simulink model "ControlSystem"  (R2024b)
settings: Solver=FixedStepAuto  StartTime=0.0  StopTime=80  RelTol=1e-3  EnableMultiTasking=on
values from neighbouring files (symbols this model uses):
  A_ESO_d = [1-l1_ESO_d, delta_t-l1_ESO_d*delta_t, 1/2 * delta_t^2 - 1/2 * l1_ESO_d*delta_t^2 ... (first row only)    [ControlSystem_Vars.m]
  A_kalman = [1 delta_t ... (first row only)    [AttitudePlayground_Vars.m]    (also in ControlSystem_Vars.m)
  A_MESO_d = A_o_d - l_MESO_d*C_o_d*A_o_d    [ControlSystem_Vars.m]
  A_O_d = A_m_dlqr - l_o_d*c_m_dlqr*A_m_dlqr    [ControlSystem_Vars.m]
  acc_sigma = 0.2 * calc_sigma(acc_pp)    [AttitudePlayground_Vars.m]    (also in ControlSystem_Vars.m)
  amfitrack_time = 1    [ControlSystem_Vars.m]
  b0 = 1.025    [ControlSystem_Vars.m]
  b_ESO_d = [1/2*b0*delta_t^2 - l1_ESO_d*b0*delta_t^2 ... (first row only)    [ControlSystem_Vars.m]
  B_MESO_d = B_o_d - l_MESO_d*C_o_d*B_o_d    [ControlSystem_Vars.m]
  B_O_d = b_m_dlqr - l_o_d*c_m_dlqr*b_m_dlqr    [ControlSystem_Vars.m]
  C_kalman = eye(2)    [AttitudePlayground_Vars.m]    (also in ControlSystem_Vars.m)
  delta_t = 0.01    [AttitudePlayground_Vars.m]    (also in ControlSystem_Vars.m; ParameterIdentification.m = t2 - t1)
  DLADRC_max_effort = 100-motor_bias    (= 70)    [ControlSystem_Vars.m]
  DLQR_ADRCNM_max_effort = 100-motor_bias    (= 70)    [ControlSystem_Vars.m]
  DLQR_max_effort = 100-motor_bias    (= 70)    [ControlSystem_Vars.m]
  DLQRMADRC_max_effort = 100-motor_bias    (= 70)    [ControlSystem_Vars.m]
  gyro_sigma_3d = [1*gyro_sigma, 1*gyro_sigma, gyro_sigma]    [AttitudePlayground_Vars.m]    (also in ControlSystem_Vars.m)
  k1_c_d = (1 - z_cl)^2/delta_t^2    [ControlSystem_Vars.m]
  k_c_T_dlqr = dlqr(A_m_dlqr,b_m_dlqr,Q,R)    [ControlSystem_Vars.m]
  k_d_T_dlqr_adrcnm = k_d_T_lqr    [ControlSystem_Vars.m]
  k_d_T_lqr = (e_m*c_T_d_m_lqr)\b_m_lqr    [ControlSystem_Vars.m]
  k_dlqr = k_c_T_dlqr    [ControlSystem_Vars.m]
  k_dlqr_adrcnm = dlqr(A_dlqr_adrcnm,B_dlqr_adrcnm,Q,R)    [ControlSystem_Vars.m]
  k_s_dlqr = -inv(c_T_m_lqr*inv(A_m_lqr-b_m_lqr*k_c_T_dlqr)*b_m_lqr)    [ControlSystem_Vars.m]
  k_T_d = [k1_c_d, k2_c_d]    [ControlSystem_Vars.m]
  l_ESO_d = [l1_ESO_d, l2_ESO_d, l3_ESO_d]'    [ControlSystem_Vars.m]
  l_MESO_d = acker(A_o_d',C_o_d',[z_MESO,z_MESO,z_MESO])'    [ControlSystem_Vars.m]
  l_o_d = acker(A_m_dlqr',c_m_dlqr',[z_o,z_o])'    [ControlSystem_Vars.m]
  motor_bias = 30    [ControlSystem_Vars.m]
  N = 1    [AttitudePlayground_Vars.m]    (also in ControlSystem_Vars.m = 2)
  P_0 = eye(4)    [AttitudePlayground_Vars.m]    (also in ControlSystem_Vars.m)
  q_sigma = 0.001    [AttitudePlayground_Vars.m]    (also in ControlSystem_Vars.m)
  R_kalman = diag([(calc_sigma(0.8))^2, (0.07)^2])    [AttitudePlayground_Vars.m]    (also in ControlSystem_Vars.m)
  reset_time = 20    [ControlSystem_Vars.m]
undefined symbols (not defined in the file or in its folder): Discrete, Time
libraries: simulink_extras x6, bbblueActuatorLib x4, ctrlSharedLib x1, bbblueSensorLib x1, sharedutil x1, dspstat3 x1, bbblueCommlib x1
settings Model: ExtModeTrigDuration=100  Creator=Henrik  LastModifiedBy=Henrik
settings SolverCC: PositivePriorityOrder=on
settings OptimizationCC: DefaultParameterBehavior=Inlined  EnhancedBackFolding=on  PassReuseOutputArgsAs=Individual arguments  ZeroExternalMemoryAtStartup=off  ZeroInternalMemoryAtStartup=off  MaxStackSize=64  OptimizeBlockOrder=speed  DifferentSizesBufferReuse=on  OptimizationCustomize=off  EfficientTunableParamExpr=on
settings DebuggingCC: ParameterTunabilityLossMsg=error
settings HardwareCC: ProdBitPerPointer=32  ProdBitPerSizeT=32  ProdBitPerPtrDiffT=32  ProdLargestAtomicInteger=Long  ProdLargestAtomicFloat=Double  ProdWordSize=32  ProdHWDeviceType=ARM Compatible->ARM Cortex-A (32-bit)  UseEmbeddedCoderFeatures=off
settings SFSimCC: MATLABDynamicMemAlloc=off
settings RTWCC: Description=Embedded Coder  SystemTargetFile=ert.tlc  HardwareBoard=BeagleBone Blue  TLCOptions="-aInlineSetEventsForThisBaseRateFcn=TLC_FALSE -aSuppressMultiTaskScheduler=TLC_FALSE  -aRateBasedStepFcn=0"  TemplateMakefile=ert_default_tmf  Toolchain=GNU GCC BeagleBone Blue
settings CodeAppCC: ForceParamTrailComments=on  IgnoreCustomStorageClasses=off  OperatorAnnotations=on  SimulinkDataObjDesc=on  SFDataObjDesc=on  InsertBlockDesc=on
settings ERTTargetCC: SupportNonInlinedSFcns=on  SupportVariableSizeSignals=on

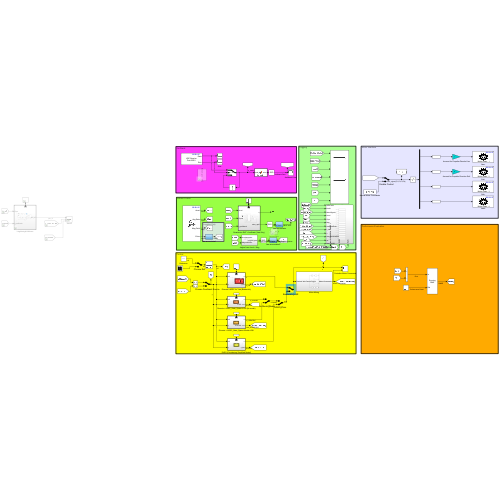
[thumbnail: Simulink's stored preview of the top-level diagram]
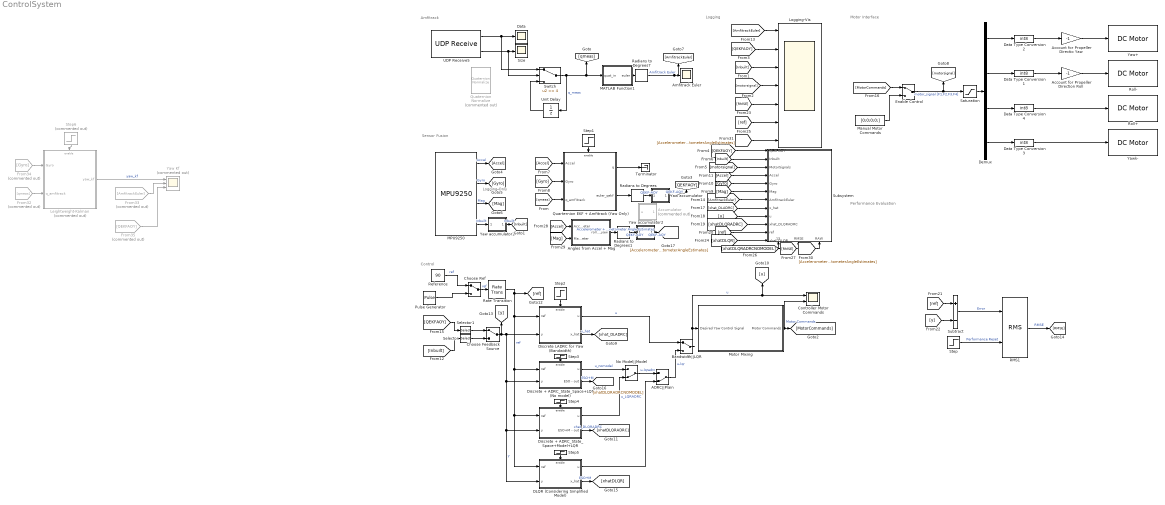
== system ControlSystem ==
  note: Performance Evaluation
  note: Control
  note: Logging Only
  note: Logging
  note: Sensor Fusion
  note: Amfitrack
  note: Motor Interface
  ADRC||Plain : ManualSwitch  CurrentSetting=0
  Account for Propeller Directio Yaw : Gain  Gain=-1  OutDataTypeStr=int8
  Account for Propeller Direction Roll : Gain  Gain=-1  OutDataTypeStr=int8
  Accumulator : Subsystem  Commented=on
  Amfitrack Euler : Scope
  Angles from Accel + Mag : Subsystem
  Bandwidth||LQR : ManualSwitch
  Choose Feedback Source : ManualSwitch
  Choose Ref : ManualSwitch
  Controller Motor Commands : Scope  NumInputPorts=2
  DLQR (Considering Simplified Model) : Subsystem
  Data : Scope
  Data Type Conversion{1..4} (4 alike) : DataTypeConversion  OutDataTypeStr=int8  SaturateOnIntegerOverflow=off  RndMeth=Floor
  Demux : Demux
  Discrete + ADRC_State_Space+LQR (No model) : Subsystem
  Discrete + ADRC_State_Space+Model+LQR : Subsystem
  Discrete LADRC for Yaw (Bandwidth) : Subsystem
  Enable Control : ManualSwitch
  From32 : From  Commented=on  GotoTag=qmeas
  From33 : From  Commented=on  GotoTag=AmfitrackEuler
  From34 : From  Commented=on  GotoTag=Gyro
  From35 : From  Commented=on  GotoTag=QEKFAOY
  Leightweight-Kalman : Subsystem  Commented=on
  Logging-Vis : Scope  NumInputPorts=7
  MATLAB Function1 : MATLAB Function  TreatAsAtomicUnit=on
  MPU9250 : bbblueSensorLib/MPU9250  OperationMode=DMP  Accel=on  AngularRate=on  Ak8963Field=on  EulerAngles=on  Quat=off  AccelRange=2G  Acceldlpf=1  GyroRange=250 dps  Gyrodlpf=1  DmpOdr=200 Hz  SampleTime=delta_t
  Manual Motor Commands : Constant  Value=[0;0;0;0;]
  Motor Mixing : Subsystem
  No Model||Model : ManualSwitch  CurrentSetting=0
  Pulse Generator : DiscretePulseGenerator  PulseType=Time based  Amplitude=90  Period=40  PulseWidth=50  PhaseDelay=25
  Quarternion EKF + Amfitrack (Yaw Only) : Subsystem
  Quaternion Normalize : sharedutil/Quaternion Normalize  Commented=on  aMode=aMode
  RMS1 : dspstat3/RMS  run=on  directionMode=Each column  dimension=1  reset_popup=Rising edge
  Radians to Degrees : simulink_extras/Transformations/Radians to Degrees
  Radians to Degrees1 : simulink_extras/Transformations/Radians to Degrees
  Radians to Degrees7 : simulink_extras/Transformations/Radians to Degrees
  Rate Transition : RateTransition  OutPortSampleTime=delta_t
  Reference : Constant  Value=90
  Roll+ : bbblueActuatorLib/DC Motor  index=3  stopaction=Free Spin  SimulateUsing=Code generation
  Roll- : bbblueActuatorLib/DC Motor  index=2  stopaction=Free Spin  SimulateUsing=Code generation
  Saturation : Saturate  UpperLimit=motor_bias + DLADRC_max_effort  LowerLimit=0
  Selector : Selector  InputPortWidth=3  IndexOptions=Index vector (dialog)  Indices=[3]  OutputSizes=1
  Selector1 : Selector  InputPortWidth=3  IndexOptions=Index vector (dialog)  Indices=[3]  OutputSizes=1
  Size : Scope
  Step : Step  Time=reset_time  SampleTime=delta_t
  Step{1..5} (5 alike) : Step  Time=amfitrack_time  SampleTime=delta_t
  Step6 : Step  Commented=on  Time=amfitrack_time  SampleTime=delta_t
  Subsystem : Subsystem
      settings: PortSchema="{\"entries\":[{\"content\":{\"sides\":[{\"content\":{\"connectorIds\":[\"In1\",\"In2\",\"In3\",\"In4\",\"In5\",\"In6\",\"In7\",\"In8\",\"In9\",\"In10\",\"In11\",\"In12\"]},\"type\":\"ConnectorPlacement.EquallySpacedRectSide\",\"uuid\":\"991a5da0-df7a-4ef3-96ef-0456b705c574\"},{\"content\":{\"side\":\"RIGHT\"},\"type\":\"ConnectorPlacement.EquallySpacedRectSide\",\"uuid\":\"461993a6-f70f-45cb-8f04-a275f01d98e3\"},{\"content\":{\"side\":\"TOP\"},\"type\":\"ConnectorPlacement.EquallySpacedRectSide\",\"uuid\":\"99c0c584-10a5-4b90-9562-b870c5806d76\"},{\"content\":{\"connectorIds\":[\"In13\",\"In14\",\"In15\"],\"side\":\"BOTTOM\"},\"type\":\"ConnectorPlacement.EquallySpacedRectSide\",\"uuid\":\"fd03c8b6-ebae-4f62-b996-a229c9f073bc\"}]},\"type\":\"ConnectorPlacement.EquallySpacedConnector\",\"uuid\":\"7a0ee6bb-fc46-401d-998f-74e037bdb036\"}],\"packageUris\":[\"http://schema.mathworks.com/mf0/Connector/R2020b\"],\"version\":\"1.0\"}"
  Subtract : Sum  Inputs=+-
  Switch : Switch  Threshold=4  SaturateOnIntegerOverflow=off  InputSameDT=off
  Terminator : Terminator
  UDP Receive5 : bbblueCommlib/UDP Receive  localURL='0.0.0.0'  localPort=25001  remoteURL='0.0.0.0'  remotePort=-1  recvBufferSize=8192  signalDatatype=double  dims=4  isVarSize=off  showBlockingTime=off  blockingTime=0  sampletime=delta_t  blockPlatform=BB BLUE
  Unit Delay : UnitDelay  InitialCondition=[1,0,0,0]'  SampleTime=-1  HasFrameUpgradeWarning=on
  Yaw Kf : Scope  Commented=on  NumInputPorts=3
  Yaw accumulator : Subsystem
  Yaw accumulator1 : Subsystem
  Yaw accumulator2 : Subsystem
  Yaw+ : bbblueActuatorLib/DC Motor  index=1  stopaction=Free Spin  SimulateUsing=Code generation
  Yawk- : bbblueActuatorLib/DC Motor  index=4  stopaction=Free Spin  SimulateUsing=Code generation
  wires:
  Unit Delay/1 -> Switch/3
  UDP Receive5/2 -> Switch/2, Size/1
  UDP Receive5/1 -> Switch/1, Data/1
  MATLAB Function1/1(euler) -> Radians to Degrees7/1
  Radians to Degrees7/1 -> Amfitrack Euler/1, [AmfitrackEuler]  "Amfitrack Euler"
  Switch/1 -> MATLAB Function1/1(quat_in), [qmeas], Unit Delay/1  "q_meas"
  [qmeas] -> Quarternion EKF + Amfitrack (Yaw Only)/3(q_amfitrack)
  Quarternion EKF + Amfitrack (Yaw Only)/1(q) -> Terminator/1
  Yaw accumulator/1(yaw_acc) -> [QEKFAOY]  "QEKF-AOY"
  [Inbuilt] -> Logging-Vis/3
  [motorsignal] -> Logging-Vis/4
  [QEKFAOY] -> Logging-Vis/2
  MPU9250/4 -> Yaw accumulator1/1(yaw)  "Inbuilt"
  MPU9250/3 -> [Mag]  "Mag"
  MPU9250/1 -> [Accel]  "Accel"
  [Accel] -> Quarternion EKF + Amfitrack (Yaw Only)/1(Accel)
  MPU9250/2 -> [Gyro]  "Gyro"
  [Gyro] -> Quarternion EKF + Amfitrack (Yaw Only)/2(Gyro)
  [QEKFAOY] -> Subsystem/1(QEKFAOY)
  [motorsignal] -> Subsystem/3(MotorSignals)
  [Inbuilt] -> Subsystem/2(Inbuilt)
  [Mag] -> Subsystem/6(Mag)
  [Gyro] -> Subsystem/5(Gyro)
  [Accel] -> Subsystem/4(Accel)
  [AmfitrackEuler] -> Logging-Vis/1
  [AmfitrackEuler] -> Subsystem/7(AmfitrackEuler)
  Account for Propeller Directio Yaw/1 -> Yaw+/1
  Data Type Conversion2/1 -> Account for Propeller Directio Yaw/1
  Data Type Conversion3/1 -> Yawk-/1
  Demux/1 -> Data Type Conversion2/1
  Demux/4 -> Data Type Conversion3/1
  Account for Propeller Direction Roll/1 -> Roll-/1
  Data Type Conversion1/1 -> Account for Propeller Direction Roll/1
  Demux/2 -> Data Type Conversion1/1
  Demux/3 -> Data Type Conversion4/1
  Data Type Conversion4/1 -> Roll+/1
  Saturation/1 -> Demux/1
  Enable Control/1 -> Saturation/1, [motorsignal]  "motor_signal [F1,F2,F3,F4]"
  Quarternion EKF + Amfitrack (Yaw Only)/2(euler_qekf) -> Radians to Degrees/1
  Manual Motor Commands/1 -> Enable Control/2
  Radians to Degrees/1 -> Yaw accumulator/1(yaw)  "QEKF-AOY"
  Yaw accumulator1/1(yaw_acc) -> [Inbuilt]  "Inbuilt"
  Bandwidth||LQR/1 -> [u], Controller Motor Commands/1, Motor Mixing/1(Desired Yaw Control Signal)  "u"
  Choose Feedback Source/1 -> DLQR (Considering Simplified Model)/2(y), Discrete + ADRC_State_Space+Model+LQR/2(y), Discrete + ADRC_State_Space+LQR (No model)/2(y), Discrete LADRC for Yaw (Bandwidth)/2(y), [y]  "y"
  Selector/1 -> Choose Feedback Source/2
  Selector1/1 -> Choose Feedback Source/1
  [Inbuilt] -> Selector/1
  [QEKFAOY] -> Selector1/1
  Rate Transition/1 -> [ref], Discrete + ADRC_State_Space+LQR (No model)/1(ref), DLQR (Considering Simplified Model)/1(ref), Discrete + ADRC_State_Space+Model+LQR/1(ref), Discrete LADRC for Yaw (Bandwidth)/1(ref)  "ref"
  Motor Mixing/1(Motor Commands) -> Controller Motor Commands/2, [MotorCommands]  "Motor Commands"
  [MotorCommands] -> Enable Control/1
  Discrete LADRC for Yaw (Bandwidth)/2(x_hat) -> [xhat_DLADRC]  "x_hat"
  [xhat_DLADRC] -> Subsystem/8(x_hat)
  [u] -> Subsystem/9(u)
  ADRC||Plain/1 -> Bandwidth||LQR/2  "u-lqr"
  Discrete LADRC for Yaw (Bandwidth)/1(u) -> Bandwidth||LQR/1  "u"
  Discrete + ADRC_State_Space+Model+LQR/2(ESO+M - out) -> [xhatDLQRADRC]  "xhat_DLQRADRC"
  [xhatDLQRADRC] -> Subsystem/10(xhat_DLQRADRC)
  [ref] -> Subsystem/11(ref)
  Subtract/1 -> RMS1/1  "Error"
  Step/1 -> RMS1/2  "Performance Reset"
  [ref] -> Subtract/1
  [y] -> Subtract/2
  RMS1/1 -> [RMSE]  "RMSE"
  [RMSE] -> Logging-Vis/5
  DLQR (Considering Simplified Model)/2(x_hat) -> [xhatDLQR]  "ESO+M"
  Discrete + ADRC_State_Space+Model+LQR/1(u) -> No Model||Model/2  "u_LQRADRC"
  DLQR (Considering Simplified Model)/1(u) -> ADRC||Plain/2
  [xhatDLQR] -> Subsystem/12(xhat_DLQR)
  Reference/1 -> Choose Ref/1  "ref"
  [ref] -> Logging-Vis/6
  Pulse Generator/1 -> Choose Ref/2
  Choose Ref/1 -> Rate Transition/1  "ref"
  Discrete + ADRC_State_Space+LQR (No model)/1(u) -> No Model||Model/1  "u_nomodel"
  No Model||Model/1 -> ADRC||Plain/1  "u-lqradrc"
  Discrete + ADRC_State_Space+LQR (No model)/2(ESO - out) -> [xhatDLQRADRCNOMODEL]  "ESO+M"
  [xhatDLQRADRCNOMODEL] -> Subsystem/13(xhatDLQRADRCNOMODEL)
  [RMSE] -> Subsystem/14(RMSE)
  [Accel] -> Angles from Accel + Mag/1(Accelerometer)
  [Mag] -> Angles from Accel + Mag/2(Magnetometer)
  Angles from Accel + Mag/1(roll,pitch,yaw) -> Radians to Degrees1/1  "Accelerometer + Magnetometer Angle Estimates"
  [AccelerometerMagnetometerAngleEstimates] -> Subsystem/15(RAW)
  [AccelerometerMagnetometerAngleEstimates] -> Logging-Vis/7
  Radians to Degrees1/1 -> Yaw accumulator2/1(yaw)  "QEKF-AOY"
  Yaw accumulator2/1(yaw_acc) -> [AccelerometerMagnetometerAngleEstimates]  "QEKF-AOY"
  Step1/1 -> Quarternion EKF + Amfitrack (Yaw Only)/Enable
  Step2/1 -> Discrete LADRC for Yaw (Bandwidth)/Enable
  Step3/1 -> Discrete + ADRC_State_Space+LQR (No model)/Enable
  Step4/1 -> Discrete + ADRC_State_Space+Model+LQR/Enable
  Step5/1 -> DLQR (Considering Simplified Model)/Enable
  From34/1 -> Leightweight-Kalman/1(Gyro)
  Step6/1 -> Leightweight-Kalman/Enable
  Leightweight-Kalman/1(yaw_kf) -> Yaw Kf/1  "yaw_kf"
  From32/1 -> Leightweight-Kalman/2(q_amfitrack)
  From33/1 -> Yaw Kf/2
  From35/1 -> Yaw Kf/3

== system ControlSystem/Accumulator ==
  u : Inport
  MATLAB Function : MATLAB Function  TreatAsAtomicUnit=on
  Unit Delay1 : UnitDelay  SampleTime=-1  HasFrameUpgradeWarning=on
  Unit Delay2 : UnitDelay  SampleTime=-1  HasFrameUpgradeWarning=on
  u_cul : Outport
  wires:
  u/1 -> Unit Delay1/1, MATLAB Function/1(u)
  Unit Delay1/1 -> MATLAB Function/2(u_prev)
  Unit Delay2/1 -> MATLAB Function/3(u_cul_prev)
  MATLAB Function/1(u_cul) -> u_cul/1, Unit Delay2/1  "u_cul"

== system ControlSystem/Angles from Accel + Mag ==
  Accelerometer : Inport
  Magnetometer : Inport  Port=2
  Demux : Demux  Outputs=3
  Demux2 : Demux  Outputs=3
  MATLAB Function : MATLAB Function  TreatAsAtomicUnit=on
  MATLAB Function1 : MATLAB Function  TreatAsAtomicUnit=on
  MATLAB Function2 : MATLAB Function  TreatAsAtomicUnit=on
  Mux : Mux  Inputs=3
  roll,pitch,yaw : Outport
  wires:
  Accelerometer/1 -> Demux/1
  Demux/1 -> MATLAB Function1/1(a_x)
  Demux/3 -> MATLAB Function1/3(a_z), MATLAB Function/2(a_z)  "az"
  Demux/2 -> MATLAB Function1/2(a_y), MATLAB Function/1(a_y)  "ay"
  Magnetometer/1 -> Demux2/1
  MATLAB Function/1(roll) -> MATLAB Function1/4(roll), Mux/1, MATLAB Function2/1(roll)  "roll"
  MATLAB Function1/1(pitch) -> Mux/2, MATLAB Function2/2(pitch)  "pitch"
  Demux2/1 -> MATLAB Function2/3(m_x)
  Demux2/2 -> MATLAB Function2/4(m_y)
  Demux2/3 -> MATLAB Function2/5(m_z)
  Mux/1 -> roll,pitch,yaw/1
  MATLAB Function2/1(yaw) -> Mux/3  "yaw"

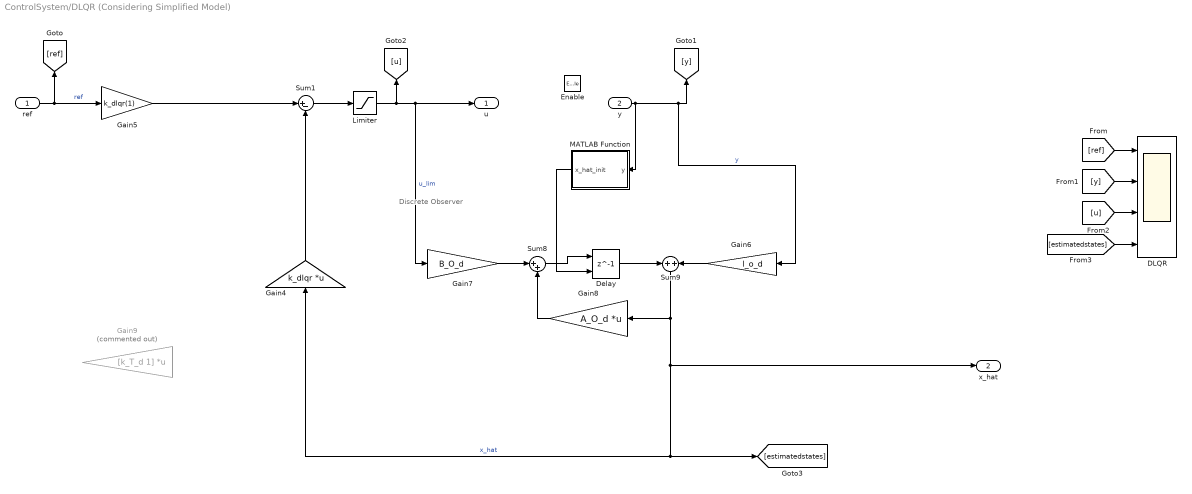
== system ControlSystem/DLQR (Considering Simplified Model) ==
  note: Discrete Observer
  ref : Inport
  y : Inport  Port=2
  Enable : EnablePort
  DLQR : Scope  NumInputPorts=4
  Delay : Delay  DelayLength=1  InitialConditionSource=Input port  SampleTime=delta_t
      settings: InputPortMap=u0,p4
  Gain4 : Gain  Gain=k_dlqr  Multiplication=Matrix(K*u)
  Gain5 : Gain  Gain=k_dlqr(1)
  Gain6 : Gain  Gain=l_o_d
  Gain7 : Gain  Gain=B_O_d
  Gain8 : Gain  Gain=A_O_d  Multiplication=Matrix(K*u)
  Gain9 : Gain  Commented=on  Gain=[k_T_d 1]  Multiplication=Matrix(K*u)
  Limiter : Saturate  UpperLimit=DLQR_max_effort  LowerLimit=-DLQR_max_effort
  MATLAB Function : MATLAB Function  TreatAsAtomicUnit=on
  Sum1 : Sum  Inputs=|+-
  Sum8 : Sum  Inputs=|++
  Sum9 : Sum  Inputs=+|+
  u : Outport
  x_hat : Outport  Port=2
  wires:
  ref/1 -> Gain5/1, [ref]  "ref"
  [ref] -> DLQR/1
  [y] -> DLQR/2
  [u] -> DLQR/3
  [estimatedstates] -> DLQR/4
  Sum1/1 -> Limiter/1
  Gain4/1 -> Sum1/2
  Gain5/1 -> Sum1/1
  Limiter/1 -> Gain7/1, u/1, [u]  "u_lim"
  Sum9/1 -> Gain4/1, [estimatedstates], x_hat/1, Gain8/1  "x_hat"
  Gain6/1 -> Sum9/2
  y/1 -> MATLAB Function/1(y), Gain6/1, [y]  "y"
  Delay/1 -> Sum9/1
  Gain7/1 -> Sum8/1
  Gain8/1 -> Sum8/2
  Sum8/1 -> Delay/1
  MATLAB Function/1(x_hat_init) -> Delay/2

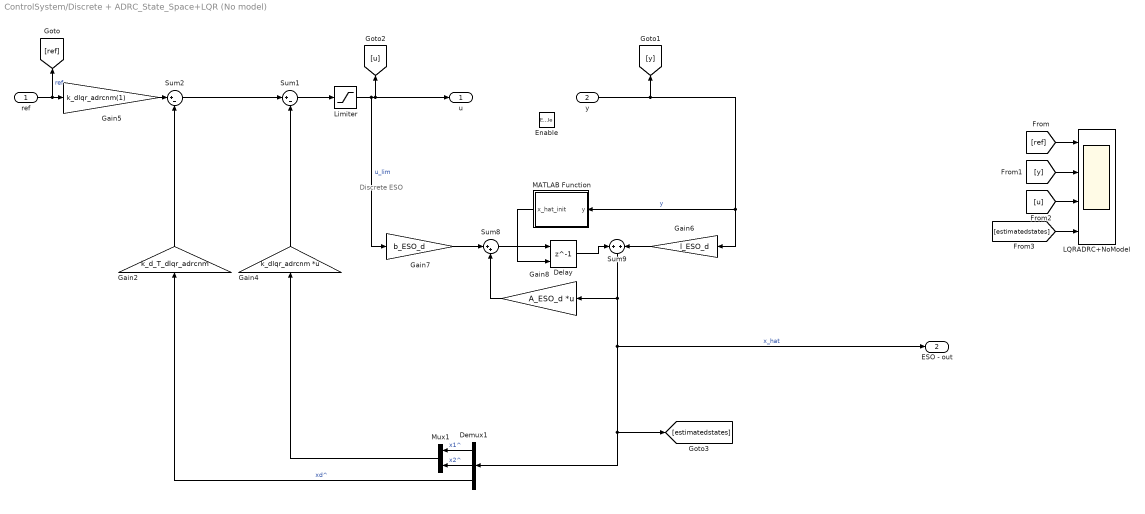
== system ControlSystem/Discrete + ADRC_State_Space+LQR (No model) ==
  note: Discrete ESO
  ref : Inport
  y : Inport  Port=2
  Enable : EnablePort
  Delay : Delay  DelayLength=1  InitialConditionSource=Input port  SampleTime=delta_t
      settings: InputPortMap=u0,p4
  Demux1 : Demux  Outputs=N+1
  Gain2 : Gain  Gain=k_d_T_dlqr_adrcnm
  Gain4 : Gain  Gain=k_dlqr_adrcnm  Multiplication=Matrix(K*u)
  Gain5 : Gain  Gain=k_dlqr_adrcnm(1)
  Gain6 : Gain  Gain=l_ESO_d
  Gain7 : Gain  Gain=b_ESO_d
  Gain8 : Gain  Gain=A_ESO_d  Multiplication=Matrix(K*u)
  LQRADRC+NoModel : Scope  NumInputPorts=4
  Limiter : Saturate  UpperLimit=DLQR_ADRCNM_max_effort  LowerLimit=-DLQR_ADRCNM_max_effort
  MATLAB Function : MATLAB Function  TreatAsAtomicUnit=on
  Mux1 : Mux  Inputs=2
  Sum1 : Sum  Inputs=|+-
  Sum2 : Sum  Inputs=|+-
  Sum8 : Sum  Inputs=|++
  Sum9 : Sum  Inputs=+|+
  u : Outport
  ESO - out : Outport  Port=2
  wires:
  ref/1 -> Gain5/1, [ref]  "ref"
  y/1 -> MATLAB Function/1(y), Gain6/1, [y]  "y"
  [ref] -> LQRADRC+NoModel/1
  [y] -> LQRADRC+NoModel/2
  [u] -> LQRADRC+NoModel/3
  [estimatedstates] -> LQRADRC+NoModel/4
  Sum1/1 -> Limiter/1
  Gain4/1 -> Sum1/2
  Gain2/1 -> Sum2/2
  Sum2/1 -> Sum1/1
  Gain5/1 -> Sum2/1
  Gain8/1 -> Sum8/2
  Delay/1 -> Sum9/1
  Gain7/1 -> Sum8/1
  Limiter/1 -> u/1, [u], Gain7/1  "u_lim"
  Sum9/1 -> Demux1/1, [estimatedstates], ESO - out/1, Gain8/1  "x_hat"
  Gain6/1 -> Sum9/2
  Demux1/1 -> Mux1/1  "x1^"
  Mux1/1 -> Gain4/1
  Demux1/2 -> Mux1/2  "x2^"
  Demux1/3 -> Gain2/1  "xd^"
  MATLAB Function/1(x_hat_init) -> Delay/2
  Sum8/1 -> Delay/1

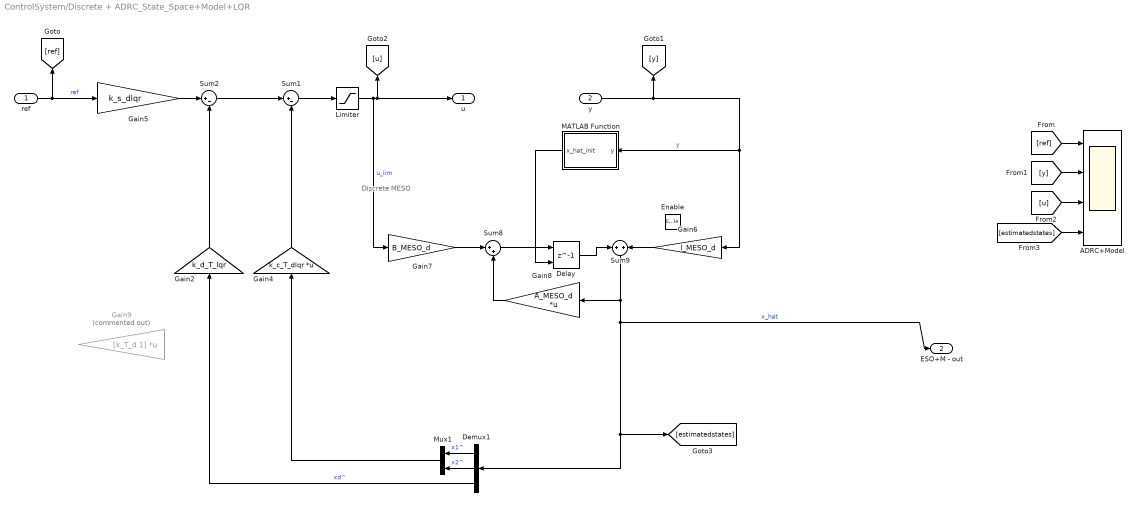
== system ControlSystem/Discrete + ADRC_State_Space+Model+LQR ==
  note: Discrete MESO
  ref : Inport
  y : Inport  Port=2
  Enable : EnablePort
  ADRC+Model : Scope  NumInputPorts=4
  Delay : Delay  DelayLength=1  InitialConditionSource=Input port  SampleTime=delta_t
      settings: InputPortMap=u0,p4
  Demux1 : Demux  Outputs=N+1
  Gain2 : Gain  Gain=k_d_T_lqr
  Gain4 : Gain  Gain=k_c_T_dlqr  Multiplication=Matrix(K*u)
  Gain5 : Gain  Gain=k_s_dlqr
  Gain6 : Gain  Gain=l_MESO_d
  Gain7 : Gain  Gain=B_MESO_d
  Gain8 : Gain  Gain=A_MESO_d  Multiplication=Matrix(K*u)
  Gain9 : Gain  Commented=on  Gain=[k_T_d 1]  Multiplication=Matrix(K*u)
  Limiter : Saturate  UpperLimit=DLQRMADRC_max_effort  LowerLimit=-DLQRMADRC_max_effort
  MATLAB Function : MATLAB Function  TreatAsAtomicUnit=on
  Mux1 : Mux  Inputs=2
  Sum1 : Sum  Inputs=|+-
  Sum2 : Sum  Inputs=|+-
  Sum8 : Sum  Inputs=|++
  Sum9 : Sum  Inputs=+|+
  u : Outport
  ESO+M - out : Outport  Port=2
  wires:
  ref/1 -> Gain5/1, [ref]  "ref"
  y/1 -> MATLAB Function/1(y), Gain6/1, [y]  "y"
  [ref] -> ADRC+Model/1
  [y] -> ADRC+Model/2
  [u] -> ADRC+Model/3
  [estimatedstates] -> ADRC+Model/4
  Sum1/1 -> Limiter/1
  Gain4/1 -> Sum1/2
  Gain2/1 -> Sum2/2
  Sum2/1 -> Sum1/1
  Gain5/1 -> Sum2/1
  Gain8/1 -> Sum8/2
  Delay/1 -> Sum9/1
  Gain7/1 -> Sum8/1
  Limiter/1 -> u/1, [u], Gain7/1  "u_lim"
  Sum9/1 -> Demux1/1, [estimatedstates], ESO+M - out/1, Gain8/1  "x_hat"
  Gain6/1 -> Sum9/2
  Demux1/1 -> Mux1/1  "x1^"
  Mux1/1 -> Gain4/1
  Demux1/2 -> Mux1/2  "x2^"
  Demux1/3 -> Gain2/1  "xd^"
  Sum8/1 -> Delay/1
  MATLAB Function/1(x_hat_init) -> Delay/2

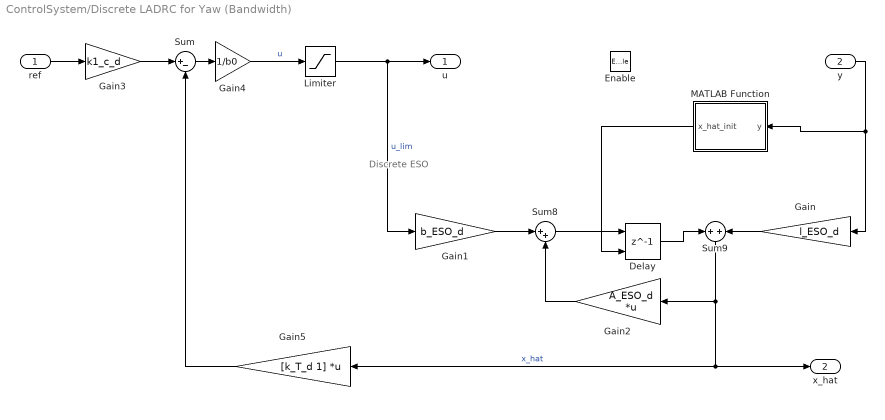
== system ControlSystem/Discrete LADRC for Yaw (Bandwidth) ==
  note: Discrete ESO
  ref : Inport
  y : Inport  Port=2
  Enable : EnablePort
  Delay : Delay  DelayLength=1  InitialConditionSource=Input port  SampleTime=delta_t
      settings: InputPortMap=u0,p4
  Gain : Gain  Gain=l_ESO_d
  Gain1 : Gain  Gain=b_ESO_d
  Gain2 : Gain  Gain=A_ESO_d  Multiplication=Matrix(K*u)
  Gain3 : Gain  Gain=k1_c_d
  Gain4 : Gain  Gain=1/b0
  Gain5 : Gain  Gain=[k_T_d 1]  Multiplication=Matrix(K*u)
  Limiter : Saturate  UpperLimit=DLADRC_max_effort  LowerLimit=-DLADRC_max_effort
  MATLAB Function : MATLAB Function  TreatAsAtomicUnit=on
  Sum : Sum  Inputs=|+-
  Sum8 : Sum  Inputs=|++
  Sum9 : Sum  Inputs=+|+
  u : Outport
  x_hat : Outport  Port=2
  wires:
  Gain1/1 -> Sum8/1
  Delay/1 -> Sum9/1
  Sum8/1 -> Delay/1
  Sum9/1 -> x_hat/1, Gain5/1, Gain2/1  "x_hat"
  Gain/1 -> Sum9/2
  Gain2/1 -> Sum8/2
  Gain4/1 -> Limiter/1  "u"
  ref/1 -> Gain3/1
  Gain3/1 -> Sum/1
  Sum/1 -> Gain4/1
  Limiter/1 -> Gain1/1, u/1  "u_lim"
  y/1 -> MATLAB Function/1(y), Gain/1
  Gain5/1 -> Sum/2
  MATLAB Function/1(x_hat_init) -> Delay/2

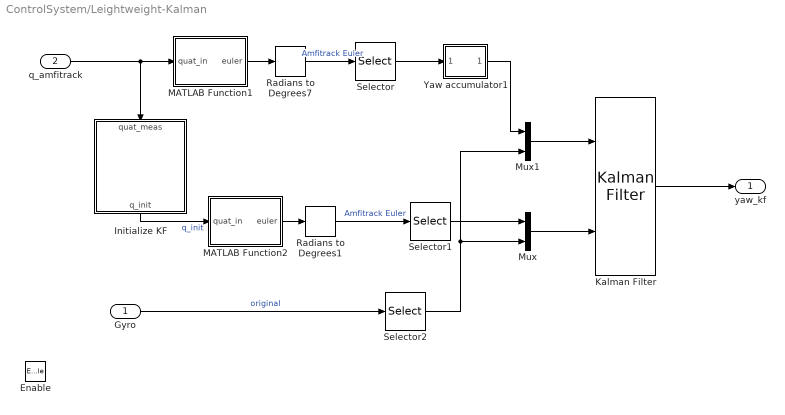
== system ControlSystem/Leightweight-Kalman ==
  Gyro : Inport
  q_amfitrack : Inport  Port=2
  Enable : EnablePort
  Initialize KF : MATLAB Function  TreatAsAtomicUnit=on
  Kalman Filter : ctrlSharedLib/Kalman Filter  TimeDomain=Discrete-Time  UseCurrentEstimator=on  ModelSource=Individual A, B, C, D matrices  ModelSourceVariable=ss(0.95,1,1,0,1)  A=A_kalman  B=1  C=C_kalman  D=0  NumberOfStates=1  NumberOfInputs=1  NumberOfOutputs=1  InitialEstimateSource=Input port  X0=0  P0=10  UseK=off  UseGH=off  NumberOfProcessNoiseInputs=1  G=1  TimeInvariantG=on  H=0  TimeInvariantH=on  Q=Q_kalman  TimeInvariantQ=on  R=R_kalman  TimeInvariantR=on  N=0  TimeInvariantN=on  AddInputPort=off  AddEnablePort=off  OutputEstimatedY=off  OutputP=off  Ts=-1
  MATLAB Function1 : MATLAB Function  TreatAsAtomicUnit=on
  MATLAB Function2 : MATLAB Function  TreatAsAtomicUnit=on
  Mux : Mux  Inputs=2
  Mux1 : Mux  Inputs=2
  Radians to Degrees1 : simulink_extras/Transformations/Radians to Degrees
  Radians to Degrees7 : simulink_extras/Transformations/Radians to Degrees
  Selector : Selector  InputPortWidth=3  IndexOptions=Index vector (dialog)  Indices=[3]  OutputSizes=1
  Selector1 : Selector  InputPortWidth=3  IndexOptions=Index vector (dialog)  Indices=[3]  OutputSizes=1
  Selector2 : Selector  InputPortWidth=3  IndexOptions=Index vector (dialog)  Indices=[3]  OutputSizes=1
  Yaw accumulator1 : Subsystem
  yaw_kf : Outport
  wires:
  Gyro/1 -> Selector2/1  "original"
  q_amfitrack/1 -> MATLAB Function1/1(quat_in), Initialize KF/1(quat_meas)
  Initialize KF/1(q_init) -> MATLAB Function2/1(quat_in)  "q_init"
  Radians to Degrees7/1 -> Selector/1  "Amfitrack Euler"
  MATLAB Function1/1(euler) -> Radians to Degrees7/1
  MATLAB Function2/1(euler) -> Radians to Degrees1/1
  Radians to Degrees1/1 -> Selector1/1  "Amfitrack Euler"
  Selector1/1 -> Mux/1
  Mux/1 -> Kalman Filter/2
  Kalman Filter/1 -> yaw_kf/1
  Selector/1 -> Yaw accumulator1/1(yaw)
  Mux1/1 -> Kalman Filter/1
  Yaw accumulator1/1(yaw_acc) -> Mux1/1
  Selector2/1 -> Mux1/2, Mux/2

== system ControlSystem/Motor Mixing ==
  Desired Yaw Control Signal : Inport
  Abs : Abs  SaturateOnIntegerOverflow=off
  Bias : Bias  Bias=motor_bias  SaturateOnIntegerOverflow=off
  Bias1 : Bias  Bias=motor_bias  SaturateOnIntegerOverflow=off
  Constant : Constant  Value=0
  Constant1 : Constant  Value=0
  If negative : Saturate  UpperLimit=0  LowerLimit=-DLADRC_max_effort
  If positive : Saturate  UpperLimit=DLADRC_max_effort  LowerLimit=0
  Mux : Mux
  Motor Commands : Outport
  wires:
  Desired Yaw Control Signal/1 -> If positive/1, If negative/1
  Mux/1 -> Motor Commands/1
  If negative/1 -> Abs/1
  If positive/1 -> Bias/1
  Abs/1 -> Bias1/1
  Constant/1 -> Mux/2
  Constant1/1 -> Mux/3
  Bias/1 -> Mux/1
  Bias1/1 -> Mux/4

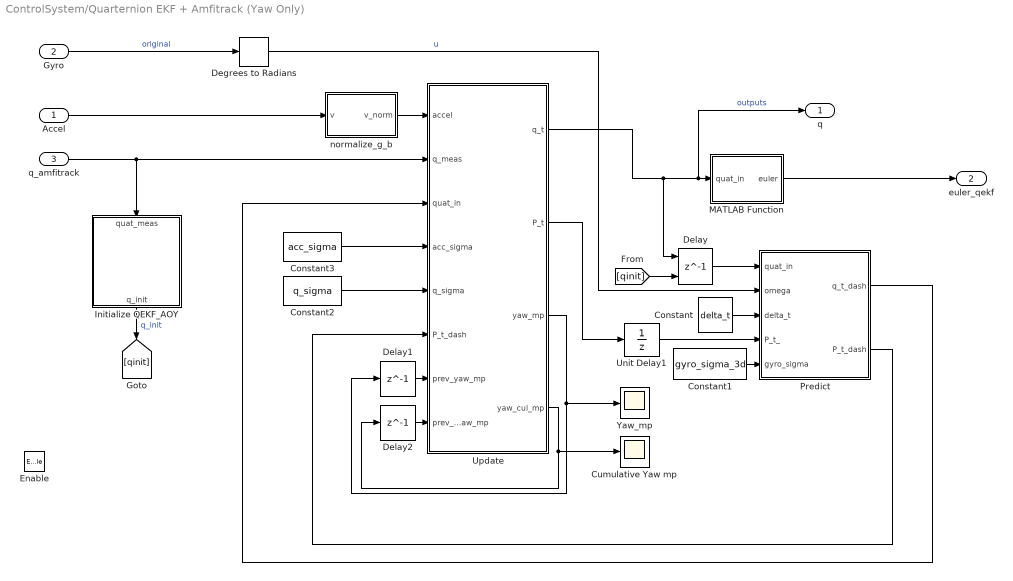
== system ControlSystem/Quarternion EKF + Amfitrack (Yaw Only) ==
  Accel : Inport
  Gyro : Inport  Port=2
  q_amfitrack : Inport  Port=3
  Enable : EnablePort
  Constant : Constant  Value=delta_t
  Constant1 : Constant  Value=gyro_sigma_3d
  Constant2 : Constant  Value=q_sigma
  Constant3 : Constant  Value=acc_sigma
  Cumulative Yaw mp : Scope
  Degrees to Radians : simulink_extras/Transformations/Degrees to Radians
  Delay : Delay  DelayLength=1  InitialConditionSource=Input port  InitialCondition=[1,0,0,0]  SampleTime=delta_t
      settings: InputPortMap=u0,p4
  Delay1 : Delay  DelayLength=1  InitialCondition=[0,0]  SampleTime=delta_t
  Delay2 : Delay  DelayLength=1  InitialCondition=[0,0]  SampleTime=delta_t
  Initialize QEKF_AOY : MATLAB Function  TreatAsAtomicUnit=on
  MATLAB Function : MATLAB Function  TreatAsAtomicUnit=on
  Predict : MATLAB Function  TreatAsAtomicUnit=on
  Unit Delay1 : UnitDelay  InitialCondition=P_0  SampleTime=delta_t  HasFrameUpgradeWarning=on
  Update : MATLAB Function  TreatAsAtomicUnit=on  SystemSampleTime=delta_t
  Yaw_mp : Scope
  normalize_g_b : MATLAB Function  TreatAsAtomicUnit=on
  q : Outport
  euler_qekf : Outport  Port=2
  wires:
  Update/1(q_t) -> Delay/1, q/1, MATLAB Function/1(quat_in)  "outputs"
  Accel/1 -> normalize_g_b/1(v)
  Constant/1 -> Predict/3(delta_t)
  Unit Delay1/1 -> Predict/4(P_t_)
  Update/2(P_t) -> Unit Delay1/1
  Predict/1(q_t_dash) -> Update/3(quat_in)
  normalize_g_b/1(v_norm) -> Update/1(accel)
  Constant3/1 -> Update/4(acc_sigma)
  Delay/1 -> Predict/1(quat_in)
  Predict/2(P_t_dash) -> Update/6(P_t_dash)
  MATLAB Function/1(euler) -> euler_qekf/1
  Degrees to Radians/1 -> Predict/2(omega)  "u"
  Gyro/1 -> Degrees to Radians/1  "original"
  Constant1/1 -> Predict/5(gyro_sigma)
  q_amfitrack/1 -> Update/2(q_meas), Initialize QEKF_AOY/1(quat_meas)
  Constant2/1 -> Update/5(q_sigma)
  Delay1/1 -> Update/7(prev_yaw_mp)
  Delay2/1 -> Update/8(prev_cul_yaw_mp)
  Update/3(yaw_mp) -> Delay1/1, Yaw_mp/1
  Update/4(yaw_cul_mp) -> Delay2/1, Cumulative Yaw mp/1
  Initialize QEKF_AOY/1(q_init) -> [qinit]  "q_init"
  [qinit] -> Delay/2

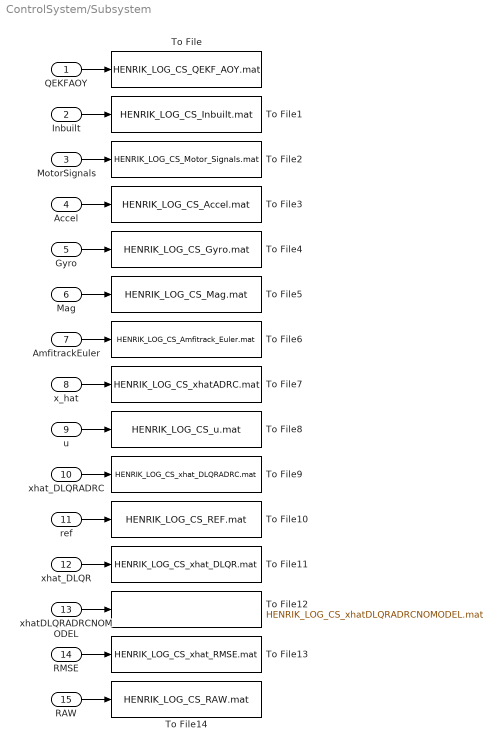
== system ControlSystem/Subsystem ==
  QEKFAOY : Inport
  Inbuilt : Inport  Port=2
  MotorSignals : Inport  Port=3
  Accel : Inport  Port=4
  Gyro : Inport  Port=5
  Mag : Inport  Port=6
  AmfitrackEuler : Inport  Port=7
  x_hat : Inport  Port=8
  u : Inport  Port=9
  xhat_DLQRADRC : Inport  Port=10
  ref : Inport  Port=11
  xhat_DLQR : Inport  Port=12
  xhatDLQRADRCNOMODEL : Inport  Port=13
  RMSE : Inport  Port=14
  RAW : Inport  Port=15
  To File : ToFile  Filename=HENRIK_LOG_CS_QEKF_AOY.mat
  To File1 : ToFile  Filename=HENRIK_LOG_CS_Inbuilt.mat
  To File10 : ToFile  Filename=HENRIK_LOG_CS_REF.mat
  To File11 : ToFile  Filename=HENRIK_LOG_CS_xhat_DLQR.mat
  To File12 : ToFile  Filename=HENRIK_LOG_CS_xhatDLQRADRCNOMODEL.mat
  To File13 : ToFile  Filename=HENRIK_LOG_CS_xhat_RMSE.mat
  To File14 : ToFile  Filename=HENRIK_LOG_CS_RAW.mat
  To File2 : ToFile  Filename=HENRIK_LOG_CS_Motor_Signals.mat
  To File3 : ToFile  Filename=HENRIK_LOG_CS_Accel.mat
  To File4 : ToFile  Filename=HENRIK_LOG_CS_Gyro.mat
  To File5 : ToFile  Filename=HENRIK_LOG_CS_Mag.mat
  To File6 : ToFile  Filename=HENRIK_LOG_CS_Amfitrack_Euler.mat
  To File7 : ToFile  Filename=HENRIK_LOG_CS_xhatADRC.mat
  To File8 : ToFile  Filename=HENRIK_LOG_CS_u.mat
  To File9 : ToFile  Filename=HENRIK_LOG_CS_xhat_DLQRADRC.mat
  wires:
  QEKFAOY/1 -> To File/1
  Inbuilt/1 -> To File1/1
  MotorSignals/1 -> To File2/1
  Mag/1 -> To File5/1
  Gyro/1 -> To File4/1
  Accel/1 -> To File3/1
  AmfitrackEuler/1 -> To File6/1
  x_hat/1 -> To File7/1
  u/1 -> To File8/1
  xhat_DLQRADRC/1 -> To File9/1
  ref/1 -> To File10/1
  xhat_DLQR/1 -> To File11/1
  xhatDLQRADRCNOMODEL/1 -> To File12/1
  RMSE/1 -> To File13/1
  RAW/1 -> To File14/1

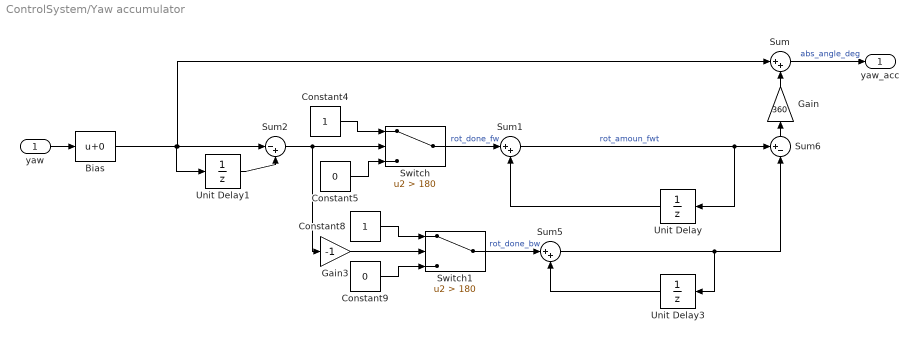
== system ControlSystem/Yaw accumulator ==
  yaw : Inport
  Bias : Bias  SaturateOnIntegerOverflow=off
  Constant4 : Constant
  Constant5 : Constant  Value=0
  Constant8 : Constant
  Constant9 : Constant  Value=0
  Gain : Gain  Gain=360
  Gain3 : Gain  Gain=-1
  Sum : Sum  Inputs=|++
  Sum1 : Sum  Inputs=|++
  Sum2 : Sum  Inputs=|-+
  Sum5 : Sum  Inputs=|++
  Sum6 : Sum  Inputs=+-|
  Switch : Switch  Criteria=u2 > Threshold  Threshold=180  SaturateOnIntegerOverflow=off  InputSameDT=off
  Switch1 : Switch  Criteria=u2 > Threshold  Threshold=180  SaturateOnIntegerOverflow=off  InputSameDT=off
  Unit Delay : UnitDelay  SampleTime=-1  HasFrameUpgradeWarning=on
  Unit Delay1 : UnitDelay  SampleTime=-1  HasFrameUpgradeWarning=on
  Unit Delay3 : UnitDelay  SampleTime=-1  HasFrameUpgradeWarning=on
  yaw_acc : Outport
  wires:
  Sum1/1 -> Unit Delay/1, Sum6/1  "rot_amoun_fwt"
  Constant5/1 -> Switch/3
  Constant8/1 -> Switch1/1
  Sum5/1 -> Unit Delay3/1, Sum6/2
  Sum6/1 -> Gain/1
  Unit Delay/1 -> Sum1/2
  Constant4/1 -> Switch/1
  yaw/1 -> Bias/1
  Unit Delay3/1 -> Sum5/2
  Switch/1 -> Sum1/1  "rot_done_fw"
  Sum2/1 -> Gain3/1, Switch/2
  Gain3/1 -> Switch1/2
  Unit Delay1/1 -> Sum2/2
  Sum/1 -> yaw_acc/1  "abs_angle_deg"
  Switch1/1 -> Sum5/1  "rot_done_bw"
  Constant9/1 -> Switch1/3
  Gain/1 -> Sum/2
  Bias/1 -> Unit Delay1/1, Sum/1, Sum2/1

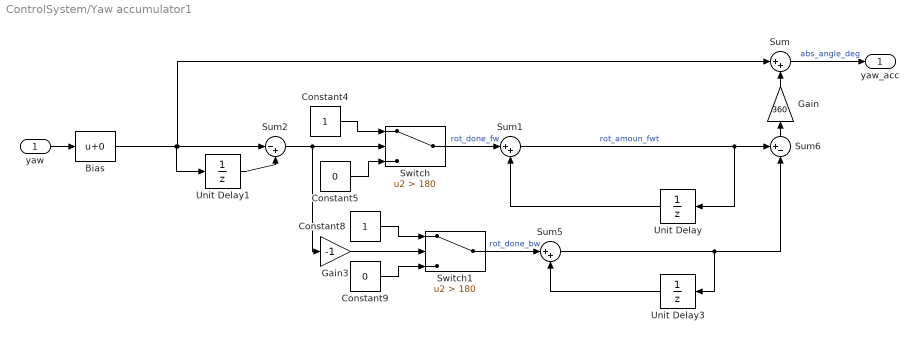
== system ControlSystem/Yaw accumulator1 ==
  yaw : Inport
  Bias : Bias  SaturateOnIntegerOverflow=off
  Constant4 : Constant
  Constant5 : Constant  Value=0
  Constant8 : Constant
  Constant9 : Constant  Value=0
  Gain : Gain  Gain=360
  Gain3 : Gain  Gain=-1
  Sum : Sum  Inputs=|++
  Sum1 : Sum  Inputs=|++
  Sum2 : Sum  Inputs=|-+
  Sum5 : Sum  Inputs=|++
  Sum6 : Sum  Inputs=+-|
  Switch : Switch  Criteria=u2 > Threshold  Threshold=180  SaturateOnIntegerOverflow=off  InputSameDT=off
  Switch1 : Switch  Criteria=u2 > Threshold  Threshold=180  SaturateOnIntegerOverflow=off  InputSameDT=off
  Unit Delay : UnitDelay  SampleTime=-1  HasFrameUpgradeWarning=on
  Unit Delay1 : UnitDelay  SampleTime=-1  HasFrameUpgradeWarning=on
  Unit Delay3 : UnitDelay  SampleTime=-1  HasFrameUpgradeWarning=on
  yaw_acc : Outport
  wires:
  Sum1/1 -> Unit Delay/1, Sum6/1  "rot_amoun_fwt"
  Constant5/1 -> Switch/3
  Constant8/1 -> Switch1/1
  Sum5/1 -> Unit Delay3/1, Sum6/2
  Sum6/1 -> Gain/1
  Unit Delay/1 -> Sum1/2
  Constant4/1 -> Switch/1
  yaw/1 -> Bias/1
  Unit Delay3/1 -> Sum5/2
  Switch/1 -> Sum1/1  "rot_done_fw"
  Sum2/1 -> Gain3/1, Switch/2
  Gain3/1 -> Switch1/2
  Unit Delay1/1 -> Sum2/2
  Sum/1 -> yaw_acc/1  "abs_angle_deg"
  Switch1/1 -> Sum5/1  "rot_done_bw"
  Constant9/1 -> Switch1/3
  Gain/1 -> Sum/2
  Bias/1 -> Unit Delay1/1, Sum/1, Sum2/1

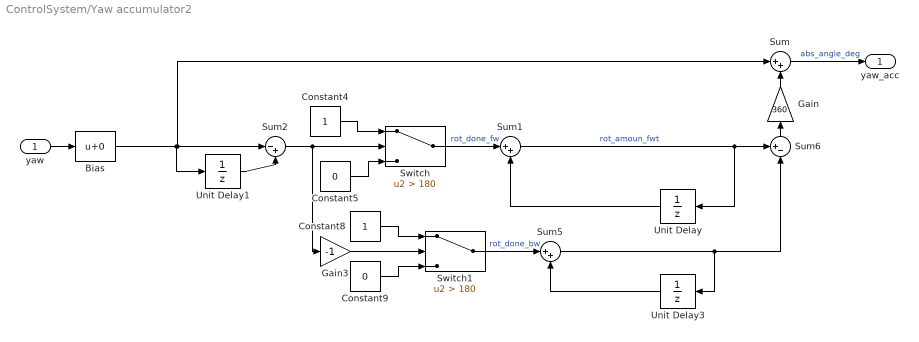
== system ControlSystem/Yaw accumulator2 ==
  yaw : Inport
  Bias : Bias  SaturateOnIntegerOverflow=off
  Constant4 : Constant
  Constant5 : Constant  Value=0
  Constant8 : Constant
  Constant9 : Constant  Value=0
  Gain : Gain  Gain=360
  Gain3 : Gain  Gain=-1
  Sum : Sum  Inputs=|++
  Sum1 : Sum  Inputs=|++
  Sum2 : Sum  Inputs=|-+
  Sum5 : Sum  Inputs=|++
  Sum6 : Sum  Inputs=+-|
  Switch : Switch  Criteria=u2 > Threshold  Threshold=180  SaturateOnIntegerOverflow=off  InputSameDT=off
  Switch1 : Switch  Criteria=u2 > Threshold  Threshold=180  SaturateOnIntegerOverflow=off  InputSameDT=off
  Unit Delay : UnitDelay  SampleTime=-1  HasFrameUpgradeWarning=on
  Unit Delay1 : UnitDelay  SampleTime=-1  HasFrameUpgradeWarning=on
  Unit Delay3 : UnitDelay  SampleTime=-1  HasFrameUpgradeWarning=on
  yaw_acc : Outport
  wires:
  Bias/1 -> Sum2/1, Sum/1, Unit Delay1/1
  Gain/1 -> Sum/2
  Constant9/1 -> Switch1/3
  Switch1/1 -> Sum5/1  "rot_done_bw"
  Sum/1 -> yaw_acc/1  "abs_angle_deg"
  Unit Delay1/1 -> Sum2/2
  Gain3/1 -> Switch1/2
  Sum2/1 -> Switch/2, Gain3/1
  Switch/1 -> Sum1/1  "rot_done_fw"
  Unit Delay3/1 -> Sum5/2
  yaw/1 -> Bias/1
  Constant4/1 -> Switch/1
  Unit Delay/1 -> Sum1/2
  Sum6/1 -> Gain/1
  Sum5/1 -> Sum6/2, Unit Delay3/1
  Constant8/1 -> Switch1/1
  Constant5/1 -> Switch/3
  Sum1/1 -> Sum6/1, Unit Delay/1  "rot_amoun_fwt"

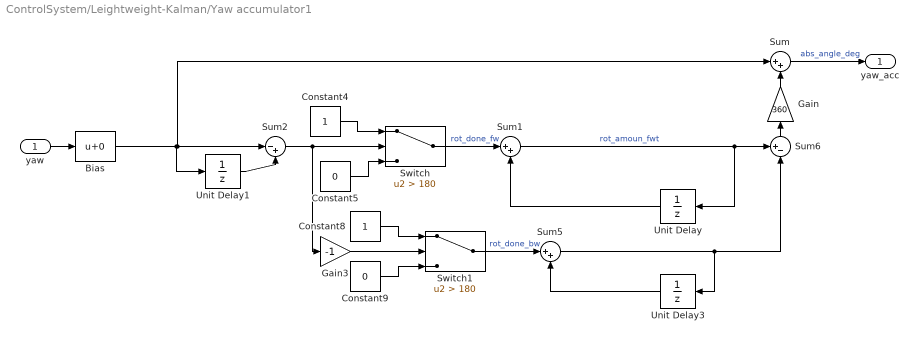
== system ControlSystem/Leightweight-Kalman/Yaw accumulator1 ==
  yaw : Inport
  Bias : Bias  SaturateOnIntegerOverflow=off
  Constant4 : Constant
  Constant5 : Constant  Value=0
  Constant8 : Constant
  Constant9 : Constant  Value=0
  Gain : Gain  Gain=360
  Gain3 : Gain  Gain=-1
  Sum : Sum  Inputs=|++
  Sum1 : Sum  Inputs=|++
  Sum2 : Sum  Inputs=|-+
  Sum5 : Sum  Inputs=|++
  Sum6 : Sum  Inputs=+-|
  Switch : Switch  Criteria=u2 > Threshold  Threshold=180  SaturateOnIntegerOverflow=off  InputSameDT=off
  Switch1 : Switch  Criteria=u2 > Threshold  Threshold=180  SaturateOnIntegerOverflow=off  InputSameDT=off
  Unit Delay : UnitDelay  SampleTime=-1  HasFrameUpgradeWarning=on
  Unit Delay1 : UnitDelay  SampleTime=-1  HasFrameUpgradeWarning=on
  Unit Delay3 : UnitDelay  SampleTime=-1  HasFrameUpgradeWarning=on
  yaw_acc : Outport
  wires:
  Sum1/1 -> Unit Delay/1, Sum6/1  "rot_amoun_fwt"
  Constant5/1 -> Switch/3
  Constant8/1 -> Switch1/1
  Sum5/1 -> Unit Delay3/1, Sum6/2
  Sum6/1 -> Gain/1
  Unit Delay/1 -> Sum1/2
  Constant4/1 -> Switch/1
  yaw/1 -> Bias/1
  Unit Delay3/1 -> Sum5/2
  Switch/1 -> Sum1/1  "rot_done_fw"
  Sum2/1 -> Gain3/1, Switch/2
  Gain3/1 -> Switch1/2
  Unit Delay1/1 -> Sum2/2
  Sum/1 -> yaw_acc/1  "abs_angle_deg"
  Switch1/1 -> Sum5/1  "rot_done_bw"
  Constant9/1 -> Switch1/3
  Gain/1 -> Sum/2
  Bias/1 -> Unit Delay1/1, Sum/1, Sum2/1

== matlab function ControlSystem/Leightweight-Kalman/MATLAB Function2 ==
  data: quat_in input; euler output
function euler = to_euler(quat_in)

q0 = quat_in(1);
q1 = quat_in(2);
q2 = quat_in(3);
q3 = quat_in(4);

roll = atan((2 * (q0*q1 + q2*q3))/(1 - 2*(q1^2 + q2^2)));
pitch = asin(2 * (q0*q2 - q1*q3));
yaw = atan2((2 * (q0*q3 + q1*q2)),(1 - 2*(q2^2 + q3^2)));

euler = [roll; pitch; yaw];

== matlab function ControlSystem/MATLAB Function1 ==
  data: quat_in input; euler output
function euler = to_euler(quat_in)

q0 = quat_in(1);
q1 = quat_in(2);
q2 = quat_in(3);
q3 = quat_in(4);

roll = atan((2 * (q0*q1 + q2*q3))/(1 - 2*(q1^2 + q2^2)));
pitch = asin(2 * (q0*q2 - q1*q3));
yaw = atan2((2 * (q0*q3 + q1*q2)),(1 - 2*(q2^2 + q3^2)));

euler = [roll; pitch; yaw];

== matlab function ControlSystem/Quarternion EKF + Amfitrack (Yaw Only)/MATLAB Function ==
  data: quat_in input; euler output
function euler = to_euler(quat_in)

q0 = quat_in(1);
q1 = quat_in(2);
q2 = quat_in(3);
q3 = quat_in(4);

roll = atan((2 * (q0*q1 + q2*q3))/(1 - 2*(q1^2 + q2^2)));
pitch = asin(2 * (q0*q2 - q1*q3));
yaw = atan2((2 * (q0*q3 + q1*q2)),(1 - 2*(q2^2 + q3^2)));

euler = [roll; pitch; yaw];

== matlab function ControlSystem/Quarternion EKF + Amfitrack (Yaw Only)/Predict ==
  data: quat_in input; q_t_dash output; omega input; delta_t input; P_t_dash output; P_t_ input; gyro_sigma input
function [q_t_dash, P_t_dash] = Predict(quat_in, omega, delta_t, P_t_, gyro_sigma)

q0 = quat_in(1);
q1 = quat_in(2);
q2 = quat_in(3);
q3 = quat_in(4);

omega_x = omega(1);
omega_y = omega(2);
omega_z = omega(3);

R_gyro = [gyro_sigma(1)^2 0 0;
          0 gyro_sigma(2)^2 0;
          0 0 gyro_sigma(3)^2;];

q0_out = q0 + delta_t/2 * (-omega_x * q1 - omega_y * q2 - omega_z * q3);
q1_out = q1 + delta_t/2 * ( omega_x * q0 - omega_y * q3 + omega_z * q2);
q2_out = q2 + delta_t/2 * ( omega_x * q3 + omega_y * q0 - omega_z * q1);
q3_out = q3 + delta_t/2 * (-omega_x * q2 + omega_y * q1 + omega_z * q0);

q_t_dash = quatnormalize([q0_out, q1_out, q2_out, q3_out]);

dt2 = delta_t/2;

F = [1  -dt2*omega_x -dt2*omega_y -dt2*omega_z;
    dt2*omega_x    1  dt2*omega_z  dt2*omega_y;
    dt2*omega_y   -dt2*omega_z   1 dt2*omega_x;
    dt2*omega_z    dt2*omega_y -dt2*omega_x  1;
    ];


W = dt2 * [-q1 -q2 -q3;
            q0 -q3  q2;
            q3  q0 -q1;
            -q2 q1  q0]; 

Q_t =  W* R_gyro * W';

P_t_dash = F * P_t_ * F' + Q_t;

== matlab function ControlSystem/Quarternion EKF + Amfitrack (Yaw Only)/Update ==
  data: accel input; q_meas input; q_t output; quat_in input; acc_sigma input; q_sigma input; P_t output; P_t_dash input; prev_yaw_mp input; prev_cul_yaw_mp input; yaw_mp output; yaw_cul_mp output
function [q_t, P_t, yaw_mp, yaw_cul_mp]   = Update(accel, q_meas, quat_in, acc_sigma, q_sigma, P_t_dash, prev_yaw_mp, prev_cul_yaw_mp)

%% Unbox function inputs
q0 = quat_in(1);
q1 = quat_in(2);
q2 = quat_in(3);
q3 = quat_in(4);

q_t_dash = [q0; q1; q2; q3];

yaw_meas_prev = prev_yaw_mp(1);
yaw_meas_cul_prev = prev_cul_yaw_mp(1);
yaw_pred_prev = prev_yaw_mp(2);
yaw_pred_cul_prev = prev_cul_yaw_mp(2);

yaw_meas = atan2((2 * (q_meas(1)*q_meas(4) + q_meas(2)*q_meas(3))),(1 - 2*(q_meas(3)^2 + q_meas(4)^2)));
yaw_pred = atan2((2 * (q0*q3 + q1*q2)),(1 - 2*(q2^2 + q3^2)));

%% Accumulate measured & predicted Yaw Angles
% Determine Change in measured and predicted Yaw angle
delta_yaw_meas = yaw_meas - yaw_meas_prev;
delta_yaw_pred = yaw_pred - yaw_pred_prev;

if delta_yaw_meas > pi
    delta_yaw_meas = delta_yaw_meas - 2*pi;
elseif delta_yaw_meas < -pi
    delta_yaw_meas = delta_yaw_meas + 2*pi;
end

yaw_meas_cul = yaw_meas_cul_prev + delta_yaw_meas;

if delta_yaw_pred > pi
    delta_yaw_pred = delta_yaw_pred - 2*pi;
elseif delta_yaw_pred < -pi
    delta_yaw_pred = delta_yaw_pred + 2*pi;
end

yaw_pred_cul = yaw_pred_cul_prev + delta_yaw_pred;

% Send them to the delay blocks for use in next update step
yaw_mp = [yaw_meas,yaw_pred];
yaw_cul_mp = [yaw_meas_cul, yaw_pred_cul];


%% Update State Estimation

% Construct measurement vector using accumulated yaw angles
z_t = [accel(1);
       accel(2);
       accel(3);
       yaw_meas_cul;
       ];

gx = 0;
gy = 0;
gz = 1;

R = [acc_sigma^2 * eye(3) zeros(3,1);
    zeros(1,3)     q_sigma^2 * eye(1)];

% Measurement Model
h = [
    2*(gx * (1/2 - q2^2 - q3^2) + gy * (q0*q3 + q1*q2) + gz * (q1*q3 - q0*q2));
    2*(gx * (q1*q2 - q0*q3) + gy * (1/2 - q1^2 - q3^2) + gz * (q0*q1 + q2*q3));
    2*(gx * (q0*q2 + q1*q3) + gy * (q2*q3 - q0*q1) + gz * (1/2 - q1^2 - q2^2));
                                    yaw_pred_cul                           ;
                                    
];

% Jacobian of Measurement Model
H = 2 * [
    gx*q0 + gy*q3 - gz*q2,  gx*q1 + gy*q2 + gz*q3, -gx*q2 + gy*q1 - gz*q0, -gx*q3 + gy*q0 + gz*q1;
   -gx*q3 + gy*q0 + gz*q1,  gx*q2 - gy*q1 + gz*q0,  gx*q1 + gy*q2 + gz*q3, -gx*q0 - gy*q3 + gz*q2;
    gx*q2 - gy*q1 + gz*q0,  gx*q3 - gy*q0 - gz*q1,  gx*q0 + gy*q3 - gz*q2,  gx*q1 + gy*q2 + gz*q3;
                                            
    0.5*[-(2*q3*(2*q2^2 + 2*q3^2 - 1))/((2*q2^2 + 2*q3^2 - 1)^2 + (2*q0*q3 + 2*q1*q2)^2), -(2*q2*(2*q2^2 + 2*q3^2 - 1))/((2*q2^2 + 2*q3^2 - 1)^2 + (2*q0*q3 + 2*q1*q2)^2), -(((2*q1)/(2*q2^2 + 2*q3^2 - 1) - (4*q2*(2*q0*q3 + 2*q1*q2))/(2*q2^2 + 2*q3^2 - 1)^2)*(2*q2^2 + 2*q3^2 - 1)^2)/((2*q2^2 + 2*q3^2 - 1)^2 + (2*q0*q3 + 2*q1*q2)^2), -(((2*q0)/(2*q2^2 + 2*q3^2 - 1) - (4*q3*(2*q0*q3 + 2*q1*q2))/(2*q2^2 + 2*q3^2 - 1)^2)*(2*q2^2 + 2*q3^2 - 1)^2)/((2*q2^2 + 2*q3^2 - 1)^2 + (2*q0*q3 + 2*q1*q2)^2)]
];

v_t = z_t - h;

S_t = H * P_t_dash * transpose(H) + R;
K_t = P_t_dash * transpose(H) * inv(S_t);

q_t = quatnormalize(transpose(q_t_dash + K_t*v_t));

P_t = (eye(4) - K_t*H) * P_t_dash;

== matlab function ControlSystem/Quarternion EKF + Amfitrack (Yaw Only)/normalize_g_b ==
  data: v input; v_norm output
function v_norm = normalize_vec(v)

v_norm = v / norm(v);

== matlab function ControlSystem/Quarternion EKF + Amfitrack (Yaw Only)/Initialize QEKF_AOY ==
  data: quat_meas input; q_init output
function q_init = calc_init_q(quat_meas)

q0 = quat_meas(1);
q1 = quat_meas(2);
q2 = quat_meas(3);
q3 = quat_meas(4);


yaw_init_rad = atan2((2 * (q0*q3 + q1*q2)),(1 - 2*(q2^2 + q3^2)));
q_init = [cos(yaw_init_rad/2), 0, 0, sin(yaw_init_rad/2)];

== matlab function ControlSystem/Angles from Accel + Mag/MATLAB Function ==
  data: a_y input; roll output; a_z input
function roll = calc_roll(a_y, a_z)

roll = atan(a_y / a_z);

== matlab function ControlSystem/Accumulator/MATLAB Function ==
  data: u input; u_cul output; u_prev input; u_cul_prev input
function u_cul = accu(u, u_prev, u_cul_prev)
delta_u = u - u_prev;


if delta_u > pi
    delta_u = delta_u - 2*pi;
elseif delta_u < -pi
    delta_u = delta_u + 2*pi;
end

u_cul = u_cul_prev + delta_u;

== matlab function ControlSystem/Angles from Accel + Mag/MATLAB Function1 ==
  data: a_x input; a_y input; pitch output; a_z input; roll input
function pitch = calc_pitch(a_x, a_y, a_z, roll)

pitch = atan(-a_x / (a_y * sin(roll) + a_z * cos(roll)));

== matlab function ControlSystem/Angles from Accel + Mag/MATLAB Function2 ==
  data: roll input; pitch input; m_x input; yaw output; m_y input; m_z input
function yaw = calc_yaw(roll, pitch, m_x, m_y, m_z)
    % Adjust for roll
    m_x2 = m_x * cos(pitch) + m_z * sin(pitch);
    m_y2 = m_x * sin(roll) * sin(pitch) + m_y * cos(roll) - m_z * sin(roll) * cos(pitch);
    % Calculate yaw
    yaw = atan2(-m_y2, m_x2);



%function yaw = calc_yaw(a_x, pitch, roll, m_x, m_y, m_z)

%m_y2 = m_z * sin(roll) - m_y * cos(roll);
%m_z2 = m_y * sin(roll) - m_z * cos(roll);
%m_x2 = m_x * cos(pitch) + m_z2 * sin(pitch);
%yaw = atan(m_y2/m_x2);

%yaw = atan(-a_x / (m_x*cos(roll)) + ...
%            m_y * sin(roll) * sin(pitch) + ...
%            m_z * cos(roll)  *sin(pitch));

== matlab function ControlSystem/Discrete + ADRC_State_Space+LQR (No model)/MATLAB Function ==
  data: y input; x_hat_init output
function x_hat_init = xhat_init(y)

x_hat_init = [y;0;0];

== matlab function ControlSystem/Discrete + ADRC_State_Space+Model+LQR/MATLAB Function ==
  data: y input; x_hat_init output
function x_hat_init = xhat_init(y)

x_hat_init = [y;0;0];

== matlab function ControlSystem/DLQR (Considering Simplified Model)/MATLAB Function ==
  data: y input; x_hat_init output
function x_hat_init = xhat_init(y)

x_hat_init = [y;0];

== matlab function ControlSystem/Discrete LADRC for Yaw (Bandwidth)/MATLAB Function ==
  data: y input; x_hat_init output
function x_hat_init = xhat_init(y)

x_hat_init = [y;0;0];

== matlab function ControlSystem/Leightweight-Kalman/Initialize KF ==
  data: quat_meas input; q_init output
function q_init = calc_init_q(quat_meas)

q0 = quat_meas(1);
q1 = quat_meas(2);
q2 = quat_meas(3);
q3 = quat_meas(4);


yaw_init_rad = atan2((2 * (q0*q3 + q1*q2)),(1 - 2*(q2^2 + q3^2)));
q_init = [cos(yaw_init_rad/2), 0, 0, sin(yaw_init_rad/2)];

== matlab function ControlSystem/Leightweight-Kalman/MATLAB Function1 ==
  data: quat_in input; euler output
function euler = to_euler(quat_in)

q0 = quat_in(1);
q1 = quat_in(2);
q2 = quat_in(3);
q3 = quat_in(4);

roll = atan((2 * (q0*q1 + q2*q3))/(1 - 2*(q1^2 + q2^2)));
pitch = asin(2 * (q0*q2 - q1*q3));
yaw = atan2((2 * (q0*q3 + q1*q2)),(1 - 2*(q2^2 + q3^2)));

euler = [roll; pitch; yaw];
